simulink model "model_c7"  (R2023b)
settings: Solver=VariableStepAuto  StartTime=0.0  StopTime=10.0  RelTol=1e-3
settings Model: Creator=gabri  LastModifiedBy=gabri

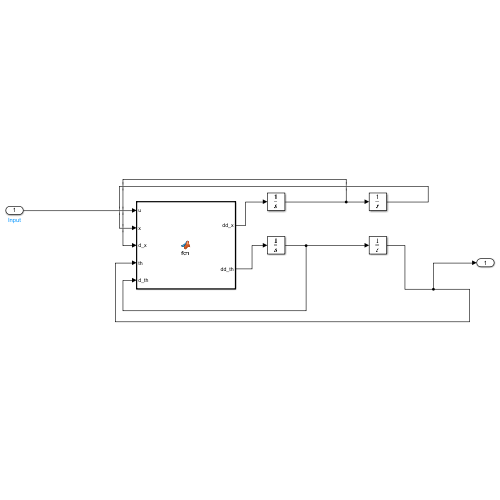
[thumbnail: Simulink's stored preview of the top-level diagram]
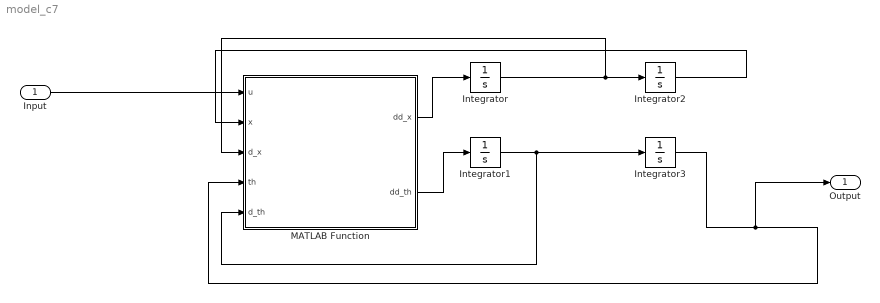
== system model_c7 ==
  Input : Inport
  Integrator{,1..3} (4 alike) : Integrator
  MATLAB Function : MATLAB Function  TreatAsAtomicUnit=on
  Output : Outport
  wires:
  MATLAB Function/2(dd_th) -> Integrator1/1
  Integrator/1 -> MATLAB Function/3(d_x), Integrator2/1
  Integrator1/1 -> Integrator3/1, MATLAB Function/5(d_th)
  Integrator3/1 -> Output/1, MATLAB Function/4(th)
  Integrator2/1 -> MATLAB Function/2(x)
  MATLAB Function/1(dd_x) -> Integrator/1
  Input/1 -> MATLAB Function/1(u)

== matlab function model_c7/MATLAB Function ==
  data: dd_x output; u input; dd_th output; x input; d_x input; th input; d_th input
function [dd_x, dd_th] = fcn(u, x, d_x, th, d_th)

l0 = 2.42;
m = 4.53;
k = 3.21;
fact = 0.71;
g = 9.81;

    %Ecuatiile
    dd_x = (l0 + x) * (d_th) * (d_th) - ((k * x) / m) + g * cos(th) - fact * d_x;
    dd_th = -(g/(l0+x)*sin(th))-(2*d_x/(l0+x))*d_th - fact*d_th + 1/(m*(l0+x)*(l0+x))*u;

end
